simulink model "sf_gfrecursive"  (Simulink 7.6)
settings: Solver=ode5  StartTime=0.0  StopTime=1  FixedStep=1  RelTol=1e-3
settings Model: Creator=The MathWorks Inc.  CovMetricSettings=dcmtr  ExtModeAutoUpdateStatusClock=off
settings OptimizationCC: BooleanDataType=off  InlineInvariantSignals=on  InitFltsAndDblsToZero=on  EfficientMapNaN2IntZero=off
settings DebuggingCC: SaveWithParameterizedLinksMsg=none  SignalResolutionControl=TryResolveAllWithWarning  SolverPrmCheckMsg=none  MultiTaskDSMMsg=warning  MultiTaskCondExecSysMsg=none  StrictBusMsg=None
settings HardwareCC: TargetUnknown=on
settings SFSimCC: SimParseCustomCode=off
settings RTWCC: IncludeERTFirstTime=on
settings GRTTargetCC: TargetFcnLib=ansi_tfl_tmw.mat

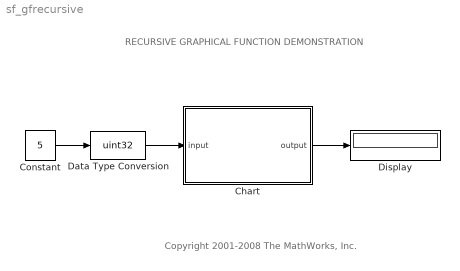
== system sf_gfrecursive ==
  note: RECURSIVE GRAPHICAL FUNCTION DEMONSTRATION
  note: Copyright 2001-2008 The MathWorks, Inc.
  Chart : Stateflow chart  TreatAsAtomicUnit=on
  Constant : Constant  Value=5
  Data Type Conversion : DataTypeConversion  OutDataTypeStr=uint32  SaturateOnIntegerOverflow=on  RndMeth=Zero
  Display : Display
  wires:
  Chart/1(output) -> Display/1
  Constant/1 -> Data Type Conversion/1
  Data Type Conversion/1 -> Chart/1(input)

== stateflow chart Chart ==
  state result = factorial(n) [function]
    (junction 5) -> (junction 4) [order 1] : [n==0]{result = 1;}
    (default) -> (junction 5)
    (junction 5) -> (junction 4) [order 2] : [n>0 && n<21]
        | {result = n*factorial(n-1);}
    (junction 5) -> (junction 4) [order 3] : /* if n >21, abort */
        | {result = 0;}
  (default) -> (junction 6) : {output = factorial(input);}
  data: n function_input uint32; result function_output uint32; input input uint32; output output uint32
